simulink library "HDL_ieee_8021513"  (R2024a)
settings: Solver=FixedStepDiscrete  StartTime=0.0  StopTime=10.0  RelTol=1e-3
undefined symbols (not defined in the file or in its folder): Add, axiWidth, channelCyclicPrefixLen, channelDataCarriers, channelEstReference, channelLUT, channelOFDMSamples, channelScramblerInit, decimatorDelay, decimatorFilter, fPHY, frequencyOffsetTimeWindow, fs, headerBitsPerFec, headerBitsPerOFDMSymbol, headerBitsPerSubcarrier, headerCyclicPrefixLen, headerDataCarriers, headerOFDMSamples, headerScramblerInit, interpolatorDelay, interpolatorFilter, leftGuard, N, ncoCarrierFrequency, ncoWordLength, numDataCarriers, oversamplingFactor, payloadBitsPerFec, payloadScramblerInit, payloadWordsPerBlock0, peakDetectorThreshold, peakDetectorWindow, preambleCyclicPrefixLen, preambleDataCarriers, preambleLUT, preambleOFDMSamples, preambleScramblerInit, QAM, rightGuard, Shift
libraries: hdlsllib x198, $bdroot x80, whdlutilities x28, whdledac x10, whdlmod x7, simulink x4, dsphdlfiltering2 x2, dsphdlsigops2 x2, commhdlcrc x2, dspsigops x2, dspstat3 x2, commdigbbndam3 x2
(part 1 of 5)
settings Model: Creator=cotti  LastModifiedBy=cotti
settings OptimizationCC: BlockReduction=off  ConditionallyExecuteInputs=off  DefaultParameterBehavior=Inlined  InheritOutputTypeSmallerThanSingle=on  ReuseModelBlockBuffer=off
settings DebuggingCC: AlgebraicLoopMsg=error  SingleTaskRateTransMsg=error
settings HardwareCC: ProdBitPerPointer=32  ProdBitPerSizeT=32  ProdBitPerPtrDiffT=32  ProdLargestAtomicFloat=None  ProdIntDivRoundTo=Undefined  ProdEndianess=Unspecified  ProdWordSize=32  ProdHWDeviceType=ASIC/FPGA->ASIC/FPGA  TargetBitPerLong=64  TargetBitPerPointer=64  TargetBitPerSizeT=64  TargetBitPerPtrDiffT=64  TargetLongLongMode=on  TargetIntDivRoundTo=Zero  TargetEndianess=LittleEndian  TargetWordSize=64  TargetHWDeviceType=Custom Processor->MATLAB Host Computer  ProdEqTarget=off
settings RTWCC: GPUComputeCapability=3.5

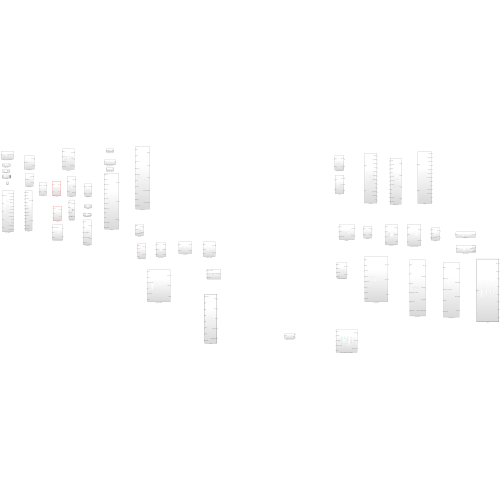
[thumbnail: Simulink's stored preview of the top-level diagram]
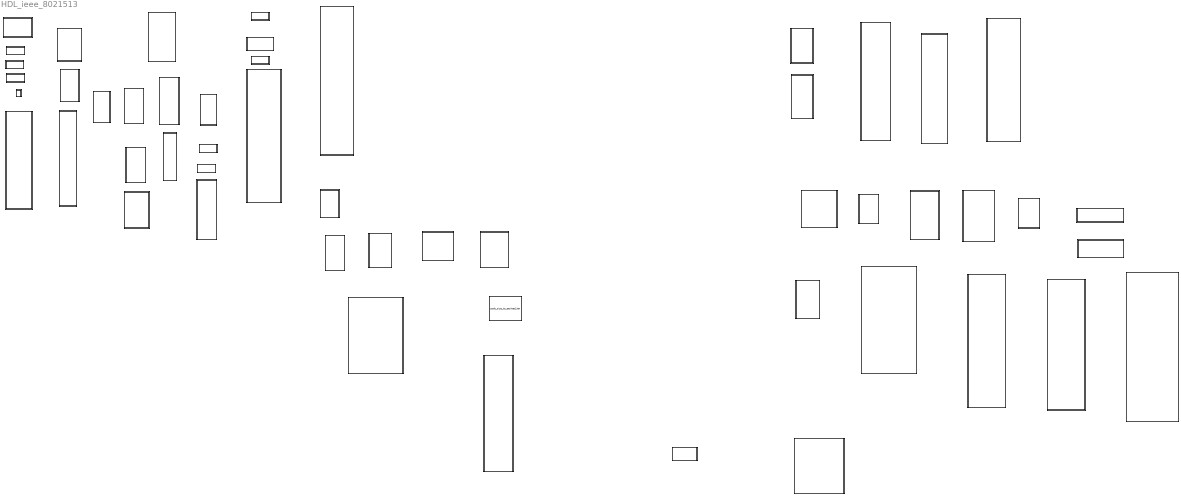
== system HDL_ieee_8021513 ==
  Buffer : Subsystem
  Deco_3a8 : Subsystem
  batid_to_bits_per_subcarrier : Subsystem
  calculate_mean_and_std : Subsystem
  channel_estimation_and_equalization : Subsystem
  channel_gen : Subsystem
  constellation_descrambler : Subsystem
  constellation_scrambler : Subsystem
  decimator : Subsystem
  downshifter : Subsystem
  falling_edge_detector : Subsystem
  frequency_upshift : Subsystem
  full_ofdm_modulator : Subsystem
  full_rx : Subsystem  TreatAsAtomicUnit=on
  full_tx : Subsystem  TreatAsAtomicUnit=on
  gnd_ctrl : Subsystem
  h_crc : Subsystem
  h_crc_rx : Subsystem
  h_gen : Subsystem
  h_remove_repetition : Subsystem
  h_repetition : Subsystem
  h_rx_full : Subsystem
  h_scrambler : Subsystem
      settings: LibrarySourceBlock=|
      | hdlsllib/Ports &
      | Subsystems/Subsystem
  h_separate : Subsystem
  header_fec : Subsystem
  header_full : Subsystem
      settings: LibrarySourceBlock=|
      | hdlsllib/Ports &
      | Subsystems/Subsystem
  interpolator : Subsystem
  ldpc_encoder : Subsystem
  next_frame_to_ready : Subsystem
  ofdm_demod : Subsystem
  ofdm_modulator : Subsystem
  ofdm_separator : Subsystem
  ofdm_symbol_sync : Subsystem
  p_scrambler : Subsystem
      settings: LibrarySourceBlock=|
      | hdlsllib/Ports &
      | Subsystems/Subsystem
  payload_full : Subsystem
  payload_rep : Subsystem
  peak_detector : Subsystem
  preamble_gen : Subsystem
  psdu_size_to_payload_len : $bdroot/payload_full/psdu_size_to_payload_len  SystemSampleTime=-1  VariantActivationTime=update diagram  AllowFlexibleInterface=on  Latency=0  AutoFrameSizeCalculation=off
  puncturer : Subsystem
  qam_demod : Subsystem
  qam_mod : Subsystem
  reduced_ldpc : Subsystem
  reg_to_variable : Subsystem
  remove_tone_mapping : Subsystem
  rising_edge_detector : Subsystem
  rx_demodulator_full : Subsystem
  rx_payload_full : Subsystem
  sync_constellation_scrambler : Subsystem
  tone_mapping : Subsystem
  valid_to_ctrl : Subsystem
  variable_to_reg : Subsystem

== system HDL_ieee_8021513/Buffer ==
  I : Inport
  O : Outport
  wires:
  I/1 -> O/1

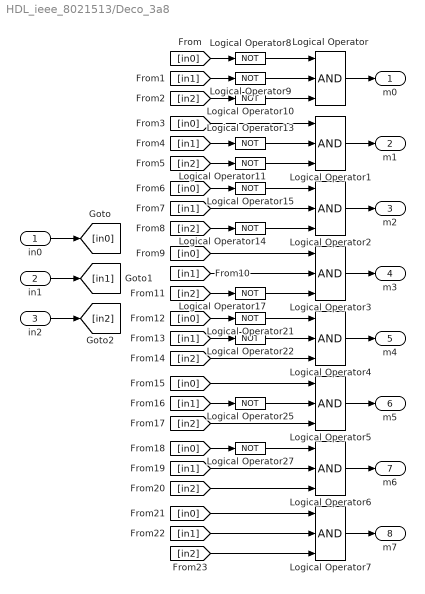
== system HDL_ieee_8021513/Deco_3a8 ==
  in0 : Inport
  in1 : Inport  Port=2
  in2 : Inport  Port=3
  Logical Operator{,1..7} (8 alike) : Logic  Inputs=3  IconShape=distinctive  AllPortsSameDT=off  OutDataTypeStr=boolean
  Logical Operator{8..11,13..15,17,21..22,25,27} (12 alike) : Logic  Operator=NOT  IconShape=distinctive  AllPortsSameDT=off  OutDataTypeStr=boolean
  m0 : Outport
  m1 : Outport  Port=2
  m2 : Outport  Port=3
  m3 : Outport  Port=4
  m4 : Outport  Port=5
  m5 : Outport  Port=6
  m6 : Outport  Port=7
  m7 : Outport  Port=8
  wires:
  Logical Operator/1 -> m0/1
  Logical Operator1/1 -> m1/1
  Logical Operator2/1 -> m2/1
  Logical Operator3/1 -> m3/1
  Logical Operator4/1 -> m4/1
  Logical Operator5/1 -> m5/1
  Logical Operator6/1 -> m6/1
  Logical Operator7/1 -> m7/1
  in0/1 -> [in0]
  in1/1 -> [in1]
  in2/1 -> [in2]
  [in0] -> Logical Operator8/1
  [in1] -> Logical Operator9/1
  [in2] -> Logical Operator10/1
  Logical Operator8/1 -> Logical Operator/1
  Logical Operator9/1 -> Logical Operator/2
  Logical Operator10/1 -> Logical Operator/3
  [in1] -> Logical Operator13/1
  [in2] -> Logical Operator11/1
  [in2] -> Logical Operator14/1
  [in0] -> Logical Operator15/1
  [in1] -> Logical Operator2/2
  [in2] -> Logical Operator17/1
  [in0] -> Logical Operator3/1
  [in1] -> Logical Operator3/2
  [in2] -> Logical Operator4/3
  [in0] -> Logical Operator21/1
  [in1] -> Logical Operator22/1
  [in2] -> Logical Operator5/3
  [in0] -> Logical Operator5/1
  [in1] -> Logical Operator25/1
  [in2] -> Logical Operator6/3
  [in0] -> Logical Operator27/1
  [in1] -> Logical Operator6/2
  [in2] -> Logical Operator7/3
  [in0] -> Logical Operator7/1
  [in1] -> Logical Operator7/2
  [in0] -> Logical Operator1/1
  Logical Operator13/1 -> Logical Operator1/2
  Logical Operator11/1 -> Logical Operator1/3
  Logical Operator15/1 -> Logical Operator2/1
  Logical Operator14/1 -> Logical Operator2/3
  Logical Operator22/1 -> Logical Operator4/2
  Logical Operator21/1 -> Logical Operator4/1
  Logical Operator17/1 -> Logical Operator3/3
  Logical Operator27/1 -> Logical Operator6/1
  Logical Operator25/1 -> Logical Operator5/2

== system HDL_ieee_8021513/batid_to_bits_per_subcarrier ==
  note: De momento, el valor de BATID va a coincidir con el valor de la cantidad de bits por subcarrier.
  note: Remember that "bat_id" is LSB first.
  bat_id : Inport
  Bit Concat : hdlsllib/Logic and Bit Operations/Bit Concat  numInputs=4
  Demux : Demux  Outputs=5
  Terminator : Terminator
  bits_per_subcarrier : Outport
  wires:
  bat_id/1 -> Demux/1
  Demux/3 -> [bat2]
  Demux/2 -> [bat1]
  Demux/4 -> [bat3]
  Demux/5 -> Terminator/1
  Demux/1 -> [bat0]
  Bit Concat/1 -> bits_per_subcarrier/1
  [bat3] -> Bit Concat/1
  [bat2] -> Bit Concat/2
  [bat1] -> Bit Concat/3
  [bat0] -> Bit Concat/4

== system HDL_ieee_8021513/calculate_mean_and_std ==
  data_in : Inport
  Delay{6..8,10..11} (5 alike) : Delay  DelayLength=1  InitialCondition=0  UseCircularBuffer=on
  Square : Math  Operator=square  SignedPower=on  RndMeth=Zero
  Subtract : Sum  Inputs=+-  OutDataTypeStr=Inherit: Same as first input
  calculate_mean_x : Subsystem
  calculate_mean_x_squared : Subsystem
  multiply by 2 : hdlsllib/Logic and Bit Operations/Bit Shift  mode=Shift Left Logical  N=1
  std : Outport
  mean : Outport  Port=2
  wires:
  Delay11/1 -> mean/1
  Subtract/1 -> Delay8/1
  Delay10/1 -> Delay11/1
  Square/1 -> Delay7/1
  Delay8/1 -> multiply by 2/1
  Delay6/1 -> Subtract/1
  calculate_mean_x/1(mean) -> Delay10/1, Square/1
  Delay7/1 -> Subtract/2
  calculate_mean_x_squared/1(mean_x_squared) -> Delay6/1
  data_in/1 -> calculate_mean_x/1(data_in), calculate_mean_x_squared/1(data_in)
  multiply by 2/1 -> std/1

== system HDL_ieee_8021513/channel_estimation_and_equalization ==
  note: Stores the estimate from Channel Estimation subsystem for each frame and perform channel equalization.
  note: Estimates the channel frequency response for each frame.
  data_in : Inport
  valid_data : Inport  Port=2
  valid_channel : Inport  Port=3
  dont_use_equalizer : Inport  Port=4
  reset : Inport  Port=5
  Channel Equalization : Subsystem
  Channel Estimation : Subsystem
  Delay{1..6,10..11,13..14} (10 alike) : Delay  DelayLength=1  InitialCondition=0
  Delay21 : Delay  InitialCondition=0
  Delay22 : Delay  InitialCondition=0
  data_out : Outport
  valid_out : Outport  Port=2
  channel_est_out : Outport  Port=3
  wires:
  reset/1 -> Channel Estimation/3(reset), Channel Equalization/6(reset)
  Delay4/1 -> channel_est_out/1
  Channel Equalization/3(channel_est_out) -> Delay4/1
  Channel Estimation/1(channel_estimate) -> Delay13/1  "channelEstimates"
  Delay22/1 -> Delay11/1
  Delay21/1 -> Delay10/1
  valid_channel/1 -> Delay2/1
  data_in/1 -> Delay1/1
  valid_data/1 -> Delay3/1
  Delay2/1 -> Channel Estimation/2(valid_in)
  Channel Estimation/2(valid_estimate) -> Delay14/1  "channelEstimatesValid"
  Delay3/1 -> Delay22/1
  Delay1/1 -> Channel Estimation/1(data_in), Delay21/1
  Channel Equalization/2(valid_out) -> Delay6/1
  Channel Equalization/1(data_out) -> Delay5/1
  Delay10/1 -> Channel Equalization/1(data_in)
  Delay11/1 -> Channel Equalization/2(valid_data)
  Delay13/1 -> Channel Equalization/3(channel_estimate_in)
  Delay14/1 -> Channel Equalization/4(valid_channel_estimate)
  Delay6/1 -> valid_out/1
  dont_use_equalizer/1 -> Channel Equalization/5(dont_use_equalizer)
  Delay5/1 -> data_out/1

== system HDL_ieee_8021513/channel_gen ==
  new_frame : Inport
  Delay : Delay  DelayLength=1  InitialCondition=0  UseCircularBuffer=on
  Direct Lookup Table (n-D) : LookupNDDirect  NumberOfTableDimensions=1  Table=channelLUT  DiagnosticForOutOfRangeInput=Error  RemoveProtectionInput=on  TableDataTypeStr=boolean
  HDL Counter : hdlsllib/Sources/HDL Counter  CountType=Count limited  CountInit=0  CountStep=1  CountMax=length(channelLUT)-1  CountFromType=Initial value  CountFrom=0  CountResetPort=off  CountLoadPort=off  CountEnbPort=on  CountDirPort=off  CountHitOutputPort=on  CountDataType=Unsigned  CountWordLen=9  CountFracLen=0  CountSampTime=1
  Logical Operator : Logic  Operator=NOT  IconShape=distinctive  AllPortsSameDT=off  OutDataTypeStr=boolean
  Logical Operator1 : Logic  Operator=OR  IconShape=distinctive  AllPortsSameDT=off  OutDataTypeStr=boolean
  Unit Delay Enabled Synchronous : hdlsllib/Discrete/Unit Delay Enabled Synchronous  InitialCondition=0.0  SampleTime=-1
  valid_to_ctrl : $bdroot/valid_to_ctrl  SystemSampleTime=-1  VariantActivationTime=update diagram  AllowFlexibleInterface=on  Latency=0  AutoFrameSizeCalculation=off
  data_out : Outport
  ctrl_out : Outport  Port=2
  wires:
  Unit Delay Enabled Synchronous/1 -> HDL Counter/1, valid_to_ctrl/1
  HDL Counter/1 -> Direct Lookup Table (n-D)/1
  Logical Operator/1 -> Unit Delay Enabled Synchronous/1
  Direct Lookup Table (n-D)/1 -> Delay/1
  valid_to_ctrl/1 -> ctrl_out/1
  Delay/1 -> data_out/1
  new_frame/1 -> Logical Operator1/1
  HDL Counter/2 -> Logical Operator1/2, Logical Operator/1
  Logical Operator1/1 -> Unit Delay Enabled Synchronous/2

== system HDL_ieee_8021513/constellation_descrambler ==
  data_in : Inport
  valid_in : Inport  Port=2
  init : Inport  Port=3
  rising_edge_detector : $bdroot/rising_edge_detector  SystemSampleTime=-1  VariantActivationTime=update diagram  AllowFlexibleInterface=on  Latency=0  AutoFrameSizeCalculation=off
  rotate_-90 : Subsystem
  sync_constellation_scrambler : $bdroot/sync_constellation_scrambler  SystemSampleTime=-1  VariantActivationTime=update diagram  AllowFlexibleInterface=on  Latency=0  AutoFrameSizeCalculation=off
  data_out : Outport
  valid_out : Outport  Port=2
  wires:
  rotate_-90/1(data_out) -> data_out/1
  rotate_-90/2(valid_out) -> valid_out/1
  sync_constellation_scrambler/2 -> rotate_-90/4(s2_in)  "s2"
  sync_constellation_scrambler/1 -> rotate_-90/3(s1_in)  "s1"
  valid_in/1 -> sync_constellation_scrambler/3, rotate_-90/2(valid_in), rising_edge_detector/1  "valid"
  init/1 -> sync_constellation_scrambler/2
  data_in/1 -> rotate_-90/1(data_in)
  rising_edge_detector/1 -> sync_constellation_scrambler/1  "start"

== system HDL_ieee_8021513/constellation_scrambler ==
  data_in : Inport
  valid_in : Inport  Port=2
  s1_in : Inport  Port=3
  s2_in : Inport  Port=4
  Delay : Delay  InitialCondition=0  UseCircularBuffer=on
  Delay1 : Delay  InitialCondition=0  UseCircularBuffer=on
  Delay2 : Delay  DelayLength=1  InitialCondition=0  UseCircularBuffer=on
  Delay3 : Delay  DelayLength=1  InitialCondition=0  UseCircularBuffer=on
  rotate : Subsystem
  data_out : Outport  VectorParamsAs1DForOutWhenUnconnected=off
  valid_out : Outport  Port=2  VectorParamsAs1DForOutWhenUnconnected=off
  wires:
  valid_in/1 -> Delay1/1  "en"
  data_in/1 -> Delay/1
  Delay/1 -> rotate/3(data_in)  "data_in"
  rotate/1(data_out) -> Delay2/1  "data_out"
  Delay1/1 -> Delay3/1
  Delay2/1 -> data_out/1  "data_out"
  Delay3/1 -> valid_out/1
  s1_in/1 -> rotate/2(s1)  "s1"
  s2_in/1 -> rotate/1(s2)  "s2"

== system HDL_ieee_8021513/decimator ==
  note: The data out from this blocks is "valid" one sample, and invalid the next.
      | This blocks makes sure that the data is valid both cycles.
      | What happens is that the ZOH might sample the signal when is valid or invalid.
  data_in : Inport
  valid_in : Inport  Port=2
  Delay{,4..7} (5 alike) : Delay  DelayLength=1  InitialCondition=0  UseCircularBuffer=on
  Delay1 : Delay  DelayLength=decimatorDelay/2  InitialCondition=0  UseCircularBuffer=on
  Delay3 : Delay  DelayLength=(decimatorDelay)*3 + 6  InitialCondition=0  UseCircularBuffer=on
  FIR Decimator : dsphdlfiltering2/FIR Decimator  Numerator=decimatorFilter.Numerator  FilterStructure=Direct form systolic  DecimationFactor=oversamplingFactor  NumCycles=1  SimulateUsing=Code generation  roundingMode=Floor  overflowMode=off  CoefficientsDataTypeStr=fixdt(1,16)  OutputDataTypeStr=fixdt(1,16,12)  ResetInputPort=off  HDLGlobalReset=off
  Logical Operator : Logic  Operator=OR  IconShape=distinctive  AllPortsSameDT=off  OutDataTypeStr=boolean
  Logical Operator1 : Logic  IconShape=distinctive  AllPortsSameDT=off  OutDataTypeStr=boolean
  Logical Operator2 : Logic  IconShape=distinctive  AllPortsSameDT=off  OutDataTypeStr=boolean
  Logical Operator3 : Logic  Operator=NOT  IconShape=distinctive  AllPortsSameDT=off  OutDataTypeStr=boolean
  Rate Transition : RateTransition  OutPortSampleTimeOpt=Multiple of input port sample time  OutPortSampleTimeMultiple=oversamplingFactor
  Rate Transition1 : RateTransition  OutPortSampleTimeOpt=Multiple of input port sample time  OutPortSampleTimeMultiple=oversamplingFactor
  Switch : Switch  Criteria=u2 ~= 0  SaturateOnIntegerOverflow=off  InputSameDT=off
  Switch1 : Switch  Criteria=u2 ~= 0  SaturateOnIntegerOverflow=off  InputSameDT=off
  falling_edge_detector : $bdroot/falling_edge_detector  SystemSampleTime=-1  VariantActivationTime=update diagram  AllowFlexibleInterface=on  Latency=0  AutoFrameSizeCalculation=off
  data_out : Outport
  valid_out : Outport  Port=2
  wires:
  Delay5/1 -> FIR Decimator/1
  Rate Transition/1 -> Delay1/1, Logical Operator1/1
  Delay4/1 -> data_out/1
  falling_edge_detector/1 -> Logical Operator3/1
  Logical Operator2/1 -> valid_out/1
  Logical Operator1/1 -> falling_edge_detector/1, Delay/1
  Logical Operator3/1 -> Logical Operator2/2
  Delay/1 -> Logical Operator2/1
  Delay7/1 -> Switch1/3
  Delay6/1 -> Switch/3
  FIR Decimator/2 -> Switch1/2, Switch1/1, Switch/2, Delay7/1  "valid_out"
  Switch1/1 -> Rate Transition/1
  FIR Decimator/1 -> Delay6/1, Switch/1  "data_out"
  Switch/1 -> Rate Transition1/1
  data_in/1 -> Delay5/1  "data_in"
  Logical Operator/1 -> FIR Decimator/2
  Delay3/1 -> Logical Operator/2
  Delay1/1 -> Logical Operator1/2
  Rate Transition1/1 -> Delay4/1
  valid_in/1 -> Delay3/1, Logical Operator/1

== system HDL_ieee_8021513/downshifter ==
  data_in : Inport
  valid_in : Inport  Port=2
  frequency_offset : Inport  Port=3
  Add : Sum  OutDataTypeStr=Inherit: Same as first input
  Constant : Constant  Value=ncoCarrierFrequency  OutDataTypeStr=int32  SampleTime=1/fs
  Delay : Delay  DelayLength=6  InitialCondition=0  UseCircularBuffer=on
  Delay1 : Delay  DelayLength=4  InitialCondition=0  UseCircularBuffer=on
  Delay{2..3,5..8} (6 alike) : Delay  DelayLength=1  InitialCondition=0  UseCircularBuffer=on
  Gain : Gain  Gain=fi(2^ncoWordLength/fs, 0, 32, 32)  ParamDataTypeStr=fixdt(0,32,32)  OutDataTypeStr=uint32  RndMeth=Round
  NCO : dsphdlsigops2/NCO  PhaseIncrementSource=Input port  PhaseIncrement=ncoPhaseIncrement  PhaseOffsetSource=Property  PhaseOffset=0  DitherSource=None  NumDitherBits=1  SamplesPerFrame=1  LUTCompress=off  ResetAction=on  Waveform=Complex exponential  PhasePort=off  SimulateUsing=Code generation  AccumulatorWL=ncoWordLength  PhaseQuantization=on  NumQuantizerAccumulatorBits=ncoQuantization  OutputDataType=Binary point scaling  OutputWL=16  OutputFL=12
  digital_carrier_receiver : Subsystem
  rising_edge_detector : $bdroot/rising_edge_detector  SystemSampleTime=-1  VariantActivationTime=update diagram  AllowFlexibleInterface=on  Latency=0  AutoFrameSizeCalculation=off
  data_out : Outport  VectorParamsAs1DForOutWhenUnconnected=off
  valid_out : Outport  Port=2  VectorParamsAs1DForOutWhenUnconnected=off
  wires:
  valid_in/1 -> Delay7/1
  Delay1/1 -> valid_out/1
  NCO/2 -> Delay1/1
  Delay3/1 -> Delay/1
  digital_carrier_receiver/1(data_out) -> data_out/1
  NCO/1 -> digital_carrier_receiver/2(ncoIn)
  Delay/1 -> digital_carrier_receiver/1(dataIn)
  data_in/1 -> Delay8/1
  Delay2/1 -> NCO/3  "valid"
  rising_edge_detector/1 -> NCO/2
  Constant/1 -> Add/1
  Add/1 -> Delay6/1
  Delay5/1 -> NCO/1  "inc"
  Delay6/1 -> Gain/1
  Gain/1 -> Delay5/1
  Delay7/1 -> rising_edge_detector/1, Delay2/1
  Delay8/1 -> Delay3/1
  frequency_offset/1 -> Add/2

== system HDL_ieee_8021513/falling_edge_detector ==
  in : Inport
  Delay : Delay  DelayLength=1  InitialCondition=0  UseCircularBuffer=on
  Logical Operator : Logic  IconShape=distinctive  AllPortsSameDT=off  OutDataTypeStr=boolean
  Logical Operator1 : Logic  Operator=NOT  IconShape=distinctive  AllPortsSameDT=off  OutDataTypeStr=boolean
  out : Outport  VectorParamsAs1DForOutWhenUnconnected=off
  wires:
  in/1 -> Logical Operator1/1, Delay/1
  Delay/1 -> Logical Operator/2
  Logical Operator/1 -> out/1
  Logical Operator1/1 -> Logical Operator/1

== system HDL_ieee_8021513/frequency_upshift ==
  data_in : Inport
  valid_in : Inport  Port=2
  reset : Inport  Port=3
  Delay : Delay  DelayLength=6  InitialCondition=0  UseCircularBuffer=on
  Delay1 : Delay  DelayLength=4  InitialCondition=0  UseCircularBuffer=on
  Delay2 : Delay  DelayLength=1  InitialCondition=0  UseCircularBuffer=on
  Delay3 : Delay  DelayLength=1  InitialCondition=0  UseCircularBuffer=on
  Mixer : Subsystem
  NCO : dsphdlsigops2/NCO  PhaseIncrementSource=Property  PhaseIncrement=ncoUpshifterPhaseIncrement  PhaseOffsetSource=Property  PhaseOffset=0  DitherSource=None  NumDitherBits=1  SamplesPerFrame=1  LUTCompress=off  ResetAction=on  Waveform=Complex exponential  PhasePort=off  SimulateUsing=Code generation  AccumulatorWL=ncoUpshifterWordLength  PhaseQuantization=off  NumQuantizerAccumulatorBits=6  OutputDataType=Binary point scaling  OutputWL=16  OutputFL=14
  data_out : Outport  VectorParamsAs1DForOutWhenUnconnected=off
  valid_out : Outport  Port=2  VectorParamsAs1DForOutWhenUnconnected=off
  wires:
  Delay2/1 -> NCO/2
  reset/1 -> NCO/1
  Delay3/1 -> Delay/1
  data_in/1 -> Delay3/1
  valid_in/1 -> Delay2/1
  NCO/1 -> Mixer/2(ncoIn)
  Mixer/1(mixedOut) -> data_out/1
  Delay/1 -> Mixer/1(dataIn)
  NCO/2 -> Delay1/1
  Delay1/1 -> valid_out/1

== system HDL_ieee_8021513/full_ofdm_modulator ==
  data_in : Inport
  valid_in : Inport  Port=2
  bits_per_subcarrier : Inport  Port=3
  init : Inport  Port=4
  new_ofdm_sym : Inport  Port=5
  cp_len : Inport  Port=6
  Delay1 : Delay  DelayLength=1  InitialCondition=0  UseCircularBuffer=on
  Logical Operator : Logic  IconShape=distinctive  AllPortsSameDT=off  OutDataTypeStr=boolean
  Logical Operator3 : Logic  IconShape=distinctive  AllPortsSameDT=off  OutDataTypeStr=boolean
  enabled_qam_and_scrambler : Subsystem  TreatAsAtomicUnit=on
  frequency_upshift : $bdroot/frequency_upshift  SystemSampleTime=-1  VariantActivationTime=update diagram  AllowFlexibleInterface=on  Latency=0  AutoFrameSizeCalculation=off
  interpolator : $bdroot/interpolator  SystemSampleTime=-1  VariantActivationTime=update diagram  AllowFlexibleInterface=on  Latency=0  AutoFrameSizeCalculation=off
  ofdm_modulator : $bdroot/ofdm_modulator  SystemSampleTime=-1  VariantActivationTime=update diagram  AllowFlexibleInterface=on  Latency=0  AutoFrameSizeCalculation=off
  rising_edge_detector : $bdroot/rising_edge_detector  SystemSampleTime=-1  VariantActivationTime=update diagram  AllowFlexibleInterface=on  Latency=0  AutoFrameSizeCalculation=off
  sync_constellation_scrambler : $bdroot/sync_constellation_scrambler  SystemSampleTime=-1  VariantActivationTime=update diagram  AllowFlexibleInterface=on  Latency=0  AutoFrameSizeCalculation=off
  data_out : Outport  VectorParamsAs1DForOutWhenUnconnected=off
  valid_out : Outport  Port=2  VectorParamsAs1DForOutWhenUnconnected=off
  ready : Outport  Port=3  VectorParamsAs1DForOutWhenUnconnected=off
  wires:
  enabled_qam_and_scrambler/4(valid_scrambler) -> Logical Operator/1
  enabled_qam_and_scrambler/6(new_out) -> sync_constellation_scrambler/1
  enabled_qam_and_scrambler/5(init_out) -> sync_constellation_scrambler/2
  enabled_qam_and_scrambler/3(cp_len_out) -> ofdm_modulator/3
  sync_constellation_scrambler/2 -> enabled_qam_and_scrambler/7(s2_in)
  sync_constellation_scrambler/1 -> enabled_qam_and_scrambler/8(s1_in)
  Logical Operator/1 -> sync_constellation_scrambler/3
  Logical Operator3/1 -> ofdm_modulator/2  "valid_new"
  enabled_qam_and_scrambler/1(data_out) -> ofdm_modulator/1  "out_new"
  Delay1/1 -> enabled_qam_and_scrambler/Enable, ready/1, Logical Operator3/1  "ready_out"
  data_in/1 -> enabled_qam_and_scrambler/1(data_in)
  init/1 -> enabled_qam_and_scrambler/4(init)
  enabled_qam_and_scrambler/2(valid_out) -> Logical Operator3/2
  ofdm_modulator/3 -> Delay1/1, Logical Operator/2
  ofdm_modulator/2 -> interpolator/2
  frequency_upshift/1 -> data_out/1
  frequency_upshift/2 -> valid_out/1
  new_ofdm_sym/1 -> enabled_qam_and_scrambler/5(new)
  bits_per_subcarrier/1 -> enabled_qam_and_scrambler/3(bits_per_subcarrier)
  interpolator/2 -> rising_edge_detector/1, frequency_upshift/2
  valid_in/1 -> enabled_qam_and_scrambler/2(valid_in)
  ofdm_modulator/1 -> interpolator/1
  interpolator/1 -> frequency_upshift/1
  rising_edge_detector/1 -> frequency_upshift/3
  cp_len/1 -> enabled_qam_and_scrambler/6(cp_len)

== system HDL_ieee_8021513/full_rx ==
  data_in : Inport
  Data Type Conversion : DataTypeConversion  OutDataTypeStr=fixdt(1,16,12)  SaturateOnIntegerOverflow=off  RndMeth=Floor
  Rate Transition{,1..2,9} (4 alike) : RateTransition  OutPortSampleTime=1/fPHY
  Rate Transition{5..8} (4 alike) : RateTransition  OutPortSampleTime=1/(4*fPHY)
  Terminator1 : Terminator
  batid_to_bits_per_subcarrier : $bdroot/batid_to_bits_per_subcarrier  SystemSampleTime=-1  VariantActivationTime=update diagram  AllowFlexibleInterface=on  Latency=0  AutoFrameSizeCalculation=off
  cpid_to_cplen : Subsystem
  h_rx_full : $bdroot/h_rx_full  SystemSampleTime=-1  VariantActivationTime=update diagram  AllowFlexibleInterface=on  Latency=0  AutoFrameSizeCalculation=off
  header_clock_x2 : Subsystem
  prepare_payload_data : Subsystem
  rx_demodulator_full : $bdroot/rx_demodulator_full  SystemSampleTime=-1  VariantActivationTime=update diagram  AllowFlexibleInterface=on  Latency=0  AutoFrameSizeCalculation=off
  rx_payload_full : $bdroot/rx_payload_full  SystemSampleTime=-1  VariantActivationTime=update diagram  AllowFlexibleInterface=on  Latency=0  AutoFrameSizeCalculation=off
  variable_to_reg : $bdroot/variable_to_reg  SystemSampleTime=-1  VariantActivationTime=update diagram  AllowFlexibleInterface=on  Latency=0  AutoFrameSizeCalculation=off
  data_out : Outport
  valid_out : Outport  Port=2
  reg0 : Outport  Port=3
  reg1 : Outport  Port=4
  reg2 : Outport  Port=5
  reg3 : Outport  Port=6
  end : Outport  Port=7
  err : Outport  Port=8
  wires:
  rx_demodulator_full/3 -> prepare_payload_data/2(valid_payload)  "valid_payload"
  rx_demodulator_full/2 -> header_clock_x2/2(valid_header)  "valid_header"
  Rate Transition9/1 -> rx_demodulator_full/5
  Rate Transition/1 -> rx_demodulator_full/4
  Rate Transition1/1 -> rx_demodulator_full/3
  Rate Transition2/1 -> rx_demodulator_full/2
  h_rx_full/6 -> variable_to_reg/6
  batid_to_bits_per_subcarrier/1 -> [payloadBitsPerSubcarrier]
  Rate Transition7/1 -> rx_payload_full/7
  variable_to_reg/1 -> reg0/1  "reg0"
  prepare_payload_data/3(last_frame) -> rx_payload_full/3
  header_clock_x2/2(start) -> h_rx_full/2
  rx_payload_full/3 -> [payloadReady]
  cpid_to_cplen/1(payload_cp_len) -> [payloadCpLen]
  h_rx_full/10 -> variable_to_reg/10
  Rate Transition5/1 -> rx_payload_full/5
  Rate Transition6/1 -> rx_payload_full/6
  h_rx_full/5 -> variable_to_reg/5
  data_in/1 -> rx_demodulator_full/1
  h_rx_full/4 -> variable_to_reg/4, Rate Transition6/1
  rx_demodulator_full/1 -> Data Type Conversion/1
  prepare_payload_data/1(dataOut) -> rx_payload_full/1
  h_rx_full/3 -> variable_to_reg/3, Rate Transition7/1
  Data Type Conversion/1 -> header_clock_x2/1(data_in), prepare_payload_data/1(data_in)
  Rate Transition8/1 -> rx_payload_full/8
  h_rx_full/11 -> variable_to_reg/11
  [payloadReady] -> prepare_payload_data/3(payload_ready)  "payload_ready"
  rx_payload_full/1 -> data_out/1
  h_rx_full/8 -> batid_to_bits_per_subcarrier/1, variable_to_reg/8
  rx_payload_full/2 -> valid_out/1
  h_rx_full/1 -> Rate Transition8/1, [psduSize], variable_to_reg/1
  h_rx_full/2 -> variable_to_reg/2
  h_rx_full/9 -> cpid_to_cplen/1(cp_id), variable_to_reg/9
  prepare_payload_data/2(valid_in) -> rx_payload_full/2  "valid_payload_to_ldpc"
  [psduSize] -> Rate Transition/1
  [payloadCpLen] -> Rate Transition2/1
  h_rx_full/13 -> err/1
  prepare_payload_data/4(new_frame) -> rx_payload_full/4
  h_rx_full/7 -> variable_to_reg/7, Rate Transition5/1
  [payloadBitsPerSubcarrier] -> Rate Transition1/1
  header_clock_x2/1(data_out) -> h_rx_full/1
  variable_to_reg/4 -> reg3/1  "reg3"
  variable_to_reg/2 -> reg1/1  "reg1"
  variable_to_reg/3 -> reg2/1  "reg2"
  h_rx_full/12 -> end/1, [header_end]  "header_ready"
  [header_end] -> Rate Transition9/1
  rx_demodulator_full/4 -> Terminator1/1  "last_frame"

== system HDL_ieee_8021513/full_tx ==
  new_frame_in : Inport
  reg0 : Inport  Port=2
  reg1 : Inport  Port=3
  reg2 : Inport  Port=4
  reg3 : Inport  Port=5
  data_in : Inport  Port=6
  valid_in : Inport  Port=7
  last_frame : Inport  Port=8
  Delay1 : Delay  DelayLength=1  InitialCondition=0  UseCircularBuffer=on
  FIFO : Subsystem  Commented=on
  Rate Transition : RateTransition  OutPortSampleTime=1/fPHY
  Sample Control Bus Selector : whdlutilities/Sample Control Bus Selector  OutputSignals=start,end,valid
  Terminator : Terminator
  Terminator1 : Terminator
  Terminator2 : Terminator
  channel_gen : $bdroot/channel_gen  SystemSampleTime=-1  VariantActivationTime=update diagram  AllowFlexibleInterface=on  Latency=0  AutoFrameSizeCalculation=off
  clock_crossing : Subsystem
  full_ofdm_modulator : $bdroot/full_ofdm_modulator  SystemSampleTime=-1  VariantActivationTime=update diagram  AllowFlexibleInterface=on  Latency=0  AutoFrameSizeCalculation=off
  header_full : $bdroot/header_full  SystemSampleTime=-1  VariantActivationTime=update diagram  AllowFlexibleInterface=on  Latency=0  AutoFrameSizeCalculation=off
      settings: LibrarySourceBlock=|
      | hdlsllib/Ports &
      | Subsystems/Subsystem
  new_frame_rate_conversion : Subsystem
  new_frame_rate_conversion1 : Subsystem
  payload_full : $bdroot/payload_full  SystemSampleTime=-1  VariantActivationTime=update diagram  AllowFlexibleInterface=on  Latency=0  AutoFrameSizeCalculation=off
  preamble_gen : $bdroot/preamble_gen  SystemSampleTime=-1  VariantActivationTime=update diagram  AllowFlexibleInterface=on  Latency=0  AutoFrameSizeCalculation=off
  reg_to_variable : $bdroot/reg_to_variable  SystemSampleTime=-1  VariantActivationTime=update diagram  AllowFlexibleInterface=on  Latency=0  AutoFrameSizeCalculation=off
  store_frame_in_ram : Subsystem
  data_out : Outport
  valid_out : Outport  Port=2
  ready : Outport  Port=3
  debug_payload : Outport  Port=4  VectorParamsAs1DForOutWhenUnconnected=off
  debug_payload_ctrl : Outport  Port=5  VectorParamsAs1DForOutWhenUnconnected=off
  wires:
  full_ofdm_modulator/3 -> store_frame_in_ram/12(ready)  "ready"
  store_frame_in_ram/6(cp_len) -> full_ofdm_modulator/6
  store_frame_in_ram/5(new) -> full_ofdm_modulator/5
  store_frame_in_ram/4(init) -> full_ofdm_modulator/4
  store_frame_in_ram/3(bits_per_subcarrier_out) -> full_ofdm_modulator/3
  store_frame_in_ram/2(valid_out) -> full_ofdm_modulator/2
  store_frame_in_ram/1(data_out) -> full_ofdm_modulator/1
  clock_crossing/1(preamble_out) -> store_frame_in_ram/1(preamble)
  clock_crossing/2(preamble_valid) -> store_frame_in_ram/2(preamble_valid)
  clock_crossing/3(channel_out) -> store_frame_in_ram/3(channel)
  clock_crossing/4(channel_valid) -> store_frame_in_ram/4(channel_valid)
  clock_crossing/5(header_out) -> store_frame_in_ram/5(header)
  clock_crossing/6(header_valid) -> store_frame_in_ram/6(header_valid)
  clock_crossing/7(payload_out) -> store_frame_in_ram/7(payload)
  clock_crossing/8(payload_valid_out) -> store_frame_in_ram/8(payload_valid)
  clock_crossing/9(payload_len_out) -> store_frame_in_ram/9(payload_len)
  clock_crossing/10(bits_per_subcarrier_out) -> store_frame_in_ram/10(bits_per_subcarrier)
  clock_crossing/11(cp_len_out) -> store_frame_in_ram/11(cp_len_in)
  Sample Control Bus Selector/2 -> channel_gen/1
  Sample Control Bus Selector/3 -> Terminator/1
  payload_full/1 -> debug_payload/1, clock_crossing/7(payload_in)
  reg_to_variable/3 -> header_full/3
  channel_gen/2 -> new_frame_rate_conversion/1(ctrl_in), clock_crossing/4(channel_ctrl)
  payload_full/5 -> clock_crossing/11(bits_per_subcarrier_in)
  reg_to_variable/9 -> payload_full/8, header_full/9
  reg_to_variable/11 -> header_full/11
  header_full/2 -> new_frame_rate_conversion1/1(ctrl_in), clock_crossing/6(header_ctrl_in)
  Rate Transition/1 -> preamble_gen/1
  header_full/1 -> clock_crossing/5(header_in)
  reg_to_variable/8 -> payload_full/5, header_full/8
  header_full/3 -> Terminator2/1
  reg_to_variable/10 -> clock_crossing/9(cp_len_in), header_full/10
  reg_to_variable/6 -> payload_full/10, header_full/6
  valid_in/1 -> payload_full/2
  channel_gen/1 -> clock_crossing/3(channel)
  new_frame_in/1 -> reg_to_variable/1
  new_frame_rate_conversion/1(new_frame) -> header_full/1
  preamble_gen/1 -> clock_crossing/1(preamble_in)
  reg1/1 -> reg_to_variable/3
  full_ofdm_modulator/2 -> valid_out/1  "valid_out"
  reg3/1 -> reg_to_variable/5
  last_frame/1 -> Delay1/1
  preamble_gen/2 -> clock_crossing/2(preamble_ctrl_in), Sample Control Bus Selector/1
  reg_to_variable/12 -> header_full/12
  new_frame_rate_conversion1/1(new_frame) -> payload_full/4  "payload_new_frame_in"
  reg2/1 -> reg_to_variable/4
  reg_to_variable/2 -> payload_full/9, header_full/2
  reg_to_variable/5 -> payload_full/6, header_full/5
  payload_full/3 -> ready/1
  payload_full/4 -> clock_crossing/10(payload_len_in)
  reg_to_variable/1 -> Rate Transition/1
  reg_to_variable/7 -> header_full/7
  data_in/1 -> payload_full/1
  Sample Control Bus Selector/1 -> Terminator1/1
  full_ofdm_modulator/1 -> data_out/1
  reg0/1 -> reg_to_variable/2
  payload_full/2 -> clock_crossing/8(payload_ctrl_in), debug_payload_ctrl/1  "payload_ctrl_out"
  reg_to_variable/4 -> payload_full/7, header_full/4
  Delay1/1 -> payload_full/3

== system HDL_ieee_8021513/gnd_ctrl ==
  Ground : Ground
  Ground1 : Ground
  Ground2 : Ground
  Sample Control Bus Creator : whdlutilities/Sample Control Bus Creator
  gnd_ctrl : Outport
  wires:
  Ground/1 -> Sample Control Bus Creator/3
  Ground1/1 -> Sample Control Bus Creator/2
  Ground2/1 -> Sample Control Bus Creator/1
  Sample Control Bus Creator/1 -> gnd_ctrl/1

== system HDL_ieee_8021513/h_crc ==
  data_in : Inport
  ctrl_in : Inport  Port=2
  General CRC Generator HDL Optimized : commhdlcrc/General CRC Generator HDL Optimized  Polynomial=headerCRCPoly  InitialState=1  DirectMethod=on  ReflectInput=off  ReflectCRCChecksum=off  FinalXORValue=0  SimulateUsing=Code generation
  Sample Control Bus Creator : whdlutilities/Sample Control Bus Creator
  Sample Control Bus Selector : whdlutilities/Sample Control Bus Selector  OutputSignals=start,end,valid
  data_out : Outport
  ctrl_out : Outport  Port=2
  wires:
  Sample Control Bus Creator/1 -> ctrl_out/1
  General CRC Generator HDL Optimized/2 -> Sample Control Bus Creator/1
  General CRC Generator HDL Optimized/3 -> Sample Control Bus Creator/2
  General CRC Generator HDL Optimized/4 -> Sample Control Bus Creator/3
  General CRC Generator HDL Optimized/1 -> data_out/1
  data_in/1 -> General CRC Generator HDL Optimized/1
  ctrl_in/1 -> Sample Control Bus Selector/1
  Sample Control Bus Selector/1 -> General CRC Generator HDL Optimized/2
  Sample Control Bus Selector/2 -> General CRC Generator HDL Optimized/3
  Sample Control Bus Selector/3 -> General CRC Generator HDL Optimized/4

== system HDL_ieee_8021513/h_crc_rx ==
  data_in : Inport
  ctrl_in : Inport  Port=2
  General CRC Syndrome Detector HDL Optimized : commhdlcrc/General CRC Syndrome Detector HDL Optimized  Polynomial=headerCRCPoly  InitialState=1  DirectMethod=on  ReflectInput=off  ReflectCRCChecksum=off  FinalXORValue=0  SimulateUsing=Code generation
  Sample Control Bus Creator : whdlutilities/Sample Control Bus Creator
  Sample Control Bus Selector : whdlutilities/Sample Control Bus Selector  OutputSignals=start,end,valid
  Switch : Switch  Criteria=u2 ~= 0  SaturateOnIntegerOverflow=off  InputSameDT=off
  Unit Delay : UnitDelay  SampleTime=-1  HasFrameUpgradeWarning=on
  data_out : Outport
  ctrl_out : Outport  Port=2  VectorParamsAs1DForOutWhenUnconnected=off
  err : Outport  Port=3  VectorParamsAs1DForOutWhenUnconnected=off
  wires:
  ctrl_in/1 -> Sample Control Bus Selector/1
  Sample Control Bus Selector/3 -> General CRC Syndrome Detector HDL Optimized/4
  Sample Control Bus Selector/2 -> General CRC Syndrome Detector HDL Optimized/3
  Sample Control Bus Selector/1 -> General CRC Syndrome Detector HDL Optimized/2
  data_in/1 -> General CRC Syndrome Detector HDL Optimized/1
  General CRC Syndrome Detector HDL Optimized/1 -> data_out/1
  General CRC Syndrome Detector HDL Optimized/2 -> Sample Control Bus Creator/1
  General CRC Syndrome Detector HDL Optimized/3 -> Switch/2, Sample Control Bus Creator/2
  General CRC Syndrome Detector HDL Optimized/4 -> Sample Control Bus Creator/3
  Sample Control Bus Creator/1 -> ctrl_out/1
  Unit Delay/1 -> Switch/3
  Switch/1 -> err/1, Unit Delay/1
  General CRC Syndrome Detector HDL Optimized/5 -> Switch/1

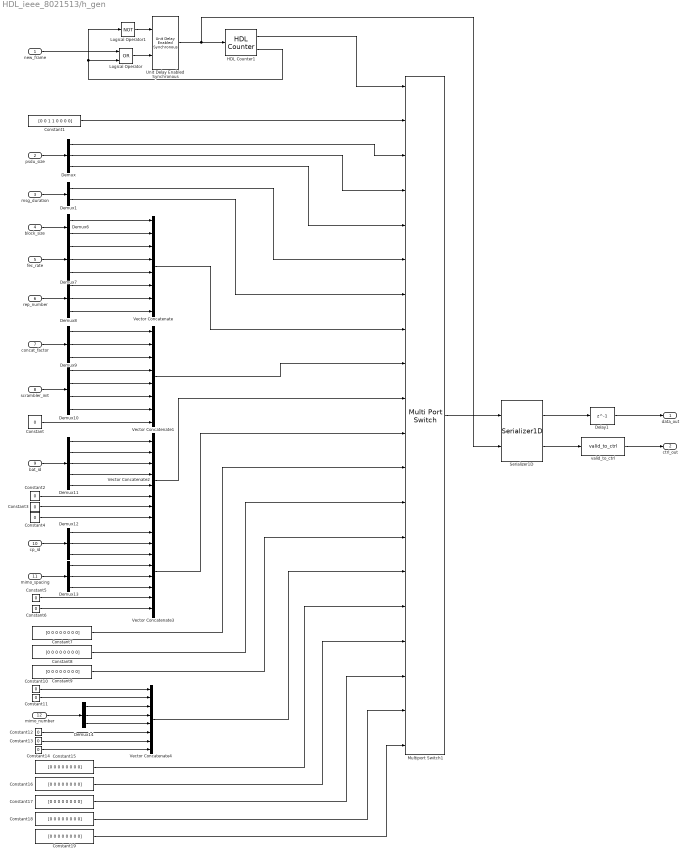
== system HDL_ieee_8021513/h_gen ==
  new_frame : Inport
  psdu_size : Inport  Port=2
  msg_duration : Inport  Port=3
  block_size : Inport  Port=4
  fec_rate : Inport  Port=5
  rep_number : Inport  Port=6
  concat_factor : Inport  Port=7
  scrambler_init : Inport  Port=8
  bat_id : Inport  Port=9
  cp_id : Inport  Port=10
  mimo_spacing : Inport  Port=11
  mimo_number : Inport  Port=12
  Constant{,2..6,10..14} (11 alike) : Constant  Value=0  OutDataTypeStr=boolean  SampleTime=-1
  Constant1 : Constant  Value=[0 0 1 1 0 0 0 0]  VectorParams1D=off  OutDataTypeStr=boolean  SampleTime=-1
  Constant{7..9,15..19} (8 alike) : Constant  Value=[0 0 0 0 0 0 0 0]  VectorParams1D=off  OutDataTypeStr=boolean  SampleTime=-1
  Delay1 : Delay  DelayLength=1  InitialCondition=0  UseCircularBuffer=on
  Demux{,7..9,12..14} (7 alike) : Demux  Outputs=3
  Demux1 : Demux  Outputs=2
  Demux10 : Demux
  Demux11 : Demux  Outputs=5
  Demux6 : Demux  Outputs=2
  HDL Counter1 : hdlsllib/Sources/HDL Counter  CountType=Count limited  CountInit=0  CountStep=1  CountMax=18  CountFromType=Initial value  CountFrom=0  CountResetPort=off  CountLoadPort=off  CountEnbPort=on  CountDirPort=off  CountHitOutputPort=on  CountDataType=Unsigned  CountWordLen=5  CountFracLen=0  CountSampTime=1
  Logical Operator : Logic  Operator=OR  IconShape=distinctive  AllPortsSameDT=off  OutDataTypeStr=boolean
  Logical Operator1 : Logic  Operator=NOT  IconShape=distinctive  AllPortsSameDT=off  OutDataTypeStr=boolean
  Multiport Switch1 : MultiPortSwitch  DataPortOrder=Zero-based contiguous  Inputs=19  zeroidx=on  OutDataTypeStr=Inherit: Same as first data input  SaturateOnIntegerOverflow=off
  Serializer1D : hdlsllib/HDL Operations/Serializer1D  Ratio=8  IdleCycles=0  validIn=on  startOut=off  validOut=on  inputDataDimensions=-1  inputSampleTime=-1  inputSignalType=auto
  Unit Delay Enabled Synchronous : hdlsllib/Discrete/Unit Delay Enabled Synchronous  InitialCondition=0.0  SampleTime=-1
  Vector Concatenate{,1..4} (5 alike) : Concatenate  NumInputs=8  Mode=Multidimensional array  ConcatenateDimension=2
  valid_to_ctrl : $bdroot/valid_to_ctrl  SystemSampleTime=-1  VariantActivationTime=update diagram  AllowFlexibleInterface=on  Latency=0  AutoFrameSizeCalculation=off
  data_out : Outport  VectorParamsAs1DForOutWhenUnconnected=off
  ctrl_out : Outport  Port=2  VectorParamsAs1DForOutWhenUnconnected=off
  wires:
  mimo_number/1 -> Demux14/1
  msg_duration/1 -> Demux1/1
  rep_number/1 -> Demux8/1
  fec_rate/1 -> Demux7/1
  block_size/1 -> Demux6/1
  concat_factor/1 -> Demux9/1
  scrambler_init/1 -> Demux10/1
  Demux/2 -> Multiport Switch1/4
  Demux/3 -> Multiport Switch1/5
  Demux1/2 -> Multiport Switch1/7
  Constant1/1 -> Multiport Switch1/2
  Vector Concatenate/1 -> Multiport Switch1/8
  Constant/1 -> Vector Concatenate1/8
  bat_id/1 -> Demux11/1
  Constant2/1 -> Vector Concatenate2/6
  Constant3/1 -> Vector Concatenate2/7
  Constant4/1 -> Vector Concatenate2/8
  Constant5/1 -> Vector Concatenate3/7
  Constant6/1 -> Vector Concatenate3/8
  Constant10/1 -> Vector Concatenate4/1
  Constant11/1 -> Vector Concatenate4/2
  Constant12/1 -> Vector Concatenate4/6
  Constant13/1 -> Vector Concatenate4/7
  Constant14/1 -> Vector Concatenate4/8
  Vector Concatenate1/1 -> Multiport Switch1/9
  Vector Concatenate2/1 -> Multiport Switch1/10
  Vector Concatenate3/1 -> Multiport Switch1/11
  Constant7/1 -> Multiport Switch1/12
  Constant8/1 -> Multiport Switch1/13
  Constant9/1 -> Multiport Switch1/14
  Vector Concatenate4/1 -> Multiport Switch1/15
  Constant15/1 -> Multiport Switch1/16
  Constant16/1 -> Multiport Switch1/17
  Constant17/1 -> Multiport Switch1/18
  Constant18/1 -> Multiport Switch1/19
  Constant19/1 -> Multiport Switch1/20
  HDL Counter1/1 -> Multiport Switch1/1
  Multiport Switch1/1 -> Serializer1D/1
  Serializer1D/1 -> Delay1/1
  new_frame/1 -> Logical Operator/1
  HDL Counter1/2 -> Logical Operator/2, Logical Operator1/1
  Logical Operator/1 -> Unit Delay Enabled Synchronous/2
  Unit Delay Enabled Synchronous/1 -> Serializer1D/2, HDL Counter1/1
  Logical Operator1/1 -> Unit Delay Enabled Synchronous/1
  Delay1/1 -> data_out/1
  Serializer1D/2 -> valid_to_ctrl/1
  valid_to_ctrl/1 -> ctrl_out/1
  Demux6/1 -> Vector Concatenate/1
  Demux6/2 -> Vector Concatenate/2
  Demux7/1 -> Vector Concatenate/3
  Demux7/2 -> Vector Concatenate/4
  Demux7/3 -> Vector Concatenate/5
  Demux8/1 -> Vector Concatenate/6
  Demux8/2 -> Vector Concatenate/7
  Demux8/3 -> Vector Concatenate/8
  Demux9/1 -> Vector Concatenate1/1
  Demux9/2 -> Vector Concatenate1/2
  Demux9/3 -> Vector Concatenate1/3
  Demux10/1 -> Vector Concatenate1/4
  Demux10/2 -> Vector Concatenate1/5
  Demux10/3 -> Vector Concatenate1/6
  Demux10/4 -> Vector Concatenate1/7
  Demux11/1 -> Vector Concatenate2/1
  Demux11/2 -> Vector Concatenate2/2
  Demux11/3 -> Vector Concatenate2/3
  Demux11/4 -> Vector Concatenate2/4
  Demux11/5 -> Vector Concatenate2/5
  Demux12/1 -> Vector Concatenate3/1
  Demux12/2 -> Vector Concatenate3/2
  Demux12/3 -> Vector Concatenate3/3
  Demux13/1 -> Vector Concatenate3/4
  Demux13/2 -> Vector Concatenate3/5
  Demux13/3 -> Vector Concatenate3/6
  Demux14/1 -> Vector Concatenate4/3
  Demux14/2 -> Vector Concatenate4/4
  Demux14/3 -> Vector Concatenate4/5
  psdu_size/1 -> Demux/1
  cp_id/1 -> Demux12/1
  mimo_spacing/1 -> Demux13/1
  Demux/1 -> Multiport Switch1/3
  Demux1/1 -> Multiport Switch1/6

== system HDL_ieee_8021513/h_remove_repetition ==
  data_in : Inport
  start_in : Inport  Port=2
  HDL Counter : hdlsllib/Sources/HDL Counter  CountType=Count limited  CountInit=0  CountStep=1  CountMax=headerBitsPerFec-1  CountFromType=Initial value  CountFrom=0  CountResetPort=on  CountLoadPort=off  CountEnbPort=on  CountDirPort=off  CountHitOutputPort=on  CountDataType=Unsigned  CountWordLen=nextpow2(headerBitsPerFec)  CountFracLen=0  CountSampTime=1
  Logical Operator : Logic  Operator=OR  AllPortsSameDT=off  OutDataTypeStr=boolean
  Sample Control Bus Creator : whdlutilities/Sample Control Bus Creator
  Switch : Switch  Criteria=u2 ~= 0  SaturateOnIntegerOverflow=off  InputSameDT=off
  Terminator : Terminator
  Unit Delay{,1..7} (8 alike) : UnitDelay  SampleTime=-1  HasFrameUpgradeWarning=on
  data_out : Outport
  ctrl_out : Outport  Port=2
  wires:
  start_in/1 -> Unit Delay3/1, Logical Operator/1, Unit Delay2/1
  HDL Counter/2 -> Logical Operator/2, Sample Control Bus Creator/2
  data_in/1 -> Unit Delay4/1
  Sample Control Bus Creator/1 -> ctrl_out/1
  Unit Delay/1 -> Switch/3
  HDL Counter/1 -> Terminator/1  "count"
  Logical Operator/1 -> Unit Delay1/1
  Unit Delay1/1 -> Switch/2
  Unit Delay2/1 -> Switch/1
  Unit Delay4/1 -> Unit Delay5/1  "data_in"
  Unit Delay3/1 -> Unit Delay6/1, HDL Counter/1  "rst"
  Switch/1 -> Unit Delay7/1, HDL Counter/2, Unit Delay/1
  Unit Delay5/1 -> data_out/1
  Unit Delay6/1 -> Sample Control Bus Creator/1
  Unit Delay7/1 -> Sample Control Bus Creator/3

== system HDL_ieee_8021513/h_repetition ==
  data_in : Inport
  ctrl_in : Inport  Port=2
  Bus Selector : BusSelector  OutputSignals=start,end,valid
  Delay{,1..4} (5 alike) : Delay  DelayLength=1  InitialCondition=0  UseCircularBuffer=on
  HDL Counter2 : hdlsllib/Sources/HDL Counter  CountType=Count limited  CountInit=headerBitsPerFec-2  CountStep=1  CountMax=headerBitsPerFec-1  CountFromType=Specify  CountFrom=0  CountResetPort=off  CountLoadPort=off  CountEnbPort=on  CountDirPort=off  CountHitOutputPort=off  CountDataType=Unsigned  CountWordLen=nextpow2(headerBitsPerOFDMSymbol)  CountFracLen=0  CountSampTime=1
  HDL Counter3 : hdlsllib/Sources/HDL Counter  CountType=Count limited  CountInit=0  CountStep=1  CountMax=headerBitsPerOFDMSymbol - headerBitsPerFec -1  CountFromType=Initial value  CountFrom=0  CountResetPort=off  CountLoadPort=off  CountEnbPort=on  CountDirPort=off  CountHitOutputPort=on  CountDataType=Unsigned  CountWordLen=nextpow2(headerBitsPerOFDMSymbol)  CountFracLen=0  CountSampTime=1
  Logical Operator : Logic  Operator=NOT  IconShape=distinctive  AllPortsSameDT=off  OutDataTypeStr=boolean
  Logical Operator1 : Logic  Operator=OR  IconShape=distinctive  AllPortsSameDT=off  OutDataTypeStr=boolean
  Logical Operator2 : Logic  Operator=NOT  IconShape=distinctive  AllPortsSameDT=off  OutDataTypeStr=boolean
  NOT : Logic  Operator=NOT  IconShape=distinctive  AllPortsSameDT=off  OutDataTypeStr=boolean
  Sample Control Bus Creator : whdlutilities/Sample Control Bus Creator
  Simple Dual Port RAM : hdlsllib/HDL RAMs/Simple Dual Port RAM  ram_size=nextpow2(headerBitsPerOFDMSymbol)
  Switch : Switch  Criteria=u2 ~= 0  SaturateOnIntegerOverflow=off  InputSameDT=off
  Switch1 : Switch  Criteria=u2 ~= 0  SaturateOnIntegerOverflow=off  InputSameDT=off
  Unit Delay Enabled Synchronous1 : hdlsllib/Discrete/Unit Delay Enabled Synchronous  InitialCondition=0.0  SampleTime=-1
  data_out : Outport  VectorParamsAs1DForOutWhenUnconnected=off
  ctrl_out : Outport  Port=2  VectorParamsAs1DForOutWhenUnconnected=off
  wires:
  Delay4/1 -> [end_out]
  Delay3/1 -> Switch1/1
  ctrl_in/1 -> Bus Selector/1
  Bus Selector/3 -> [valid], Delay3/1  "<valid>"
  Sample Control Bus Creator/1 -> ctrl_out/1
  Bus Selector/1 -> Delay/1  "<start>"
  Bus Selector/2 -> [end]  "<end>"
  Delay/1 -> Sample Control Bus Creator/1
  [end_out] -> Sample Control Bus Creator/2
  Switch1/1 -> Sample Control Bus Creator/3
  [valid] -> HDL Counter2/1  "addrB_valid"
  [valid] -> Simple Dual Port RAM/3
  HDL Counter2/1 -> Simple Dual Port RAM/2
  data_in/1 -> Delay1/1, Simple Dual Port RAM/1  "datain"
  HDL Counter3/1 -> Simple Dual Port RAM/4  "addrA"
  Unit Delay Enabled Synchronous1/1 -> HDL Counter3/1, Delay2/1
  [end] -> Logical Operator1/1
  Logical Operator1/1 -> Unit Delay Enabled Synchronous1/2
  HDL Counter3/2 -> Logical Operator1/2, NOT/1, Delay4/1
  NOT/1 -> Unit Delay Enabled Synchronous1/1
  Switch/1 -> data_out/1
  Delay2/1 -> Logical Operator2/1, Switch1/3, Logical Operator/1
  Simple Dual Port RAM/1 -> Switch/3
  Delay1/1 -> Switch/1
  Logical Operator/1 -> Switch1/2
  Logical Operator2/1 -> Switch/2

== system HDL_ieee_8021513/h_rx_full ==
  data_in : Inport
  start_in : Inport  Port=2
  Data Type Conversion : DataTypeConversion  OutDataTypeStr=int8  SaturateOnIntegerOverflow=off  RndMeth=Floor
  Data Type Conversion1 : DataTypeConversion  OutDataTypeStr=boolean  SaturateOnIntegerOverflow=off  RndMeth=Floor
  LDPC_Deco_Hc_12H : whdledac/LDPC Decoder  ParityCheckMatrix=Hc_12H  BlockSize=14  Algorithm=Min-sum  ScalingFactor=0.75  Termination=Max  SpecifyInputs=Property  NumIterations=ldpcDecoderMaxNumberIterations  MaxNumIterations=8  ParityCheckStatus=off  SimulateUsing=Code generation
  Rate Transition : RateTransition  OutPortSampleTimeOpt=Multiple of input port sample time  OutPortSampleTimeMultiple=8
  Terminator : Terminator
  h_crc_rx : $bdroot/h_crc_rx  SystemSampleTime=-1  VariantActivationTime=update diagram  AllowFlexibleInterface=on  Latency=0  AutoFrameSizeCalculation=off
  h_remove_repetition : $bdroot/h_remove_repetition  SystemSampleTime=-1  VariantActivationTime=update diagram  AllowFlexibleInterface=on  Latency=0  AutoFrameSizeCalculation=off
  h_scrambler : $bdroot/h_scrambler  SystemSampleTime=-1  VariantActivationTime=update diagram  AllowFlexibleInterface=on  Latency=0  AutoFrameSizeCalculation=off
      settings: LibrarySourceBlock=|
      | hdlsllib/Ports &
      | Subsystems/Subsystem
  h_separate : $bdroot/h_separate  SystemSampleTime=-1  VariantActivationTime=update diagram  AllowFlexibleInterface=on  Latency=0  AutoFrameSizeCalculation=off
  psdu_size : Outport
  msg_duration : Outport  Port=2
  block_size : Outport  Port=3
  fec_rate : Outport  Port=4
  rep_number : Outport  Port=5
  concat_factor : Outport  Port=6
  scrambler_init : Outport  Port=7
  bat_id : Outport  Port=8
  cp_id : Outport  Port=9
  mimo_spacing : Outport  Port=10
  mimo_number : Outport  Port=11
  end : Outport  Port=12
  err : Outport  Port=13
  wires:
  Rate Transition/1 -> err/1
  h_separate/4 -> fec_rate/1
  h_separate/1 -> psdu_size/1
  h_remove_repetition/2 -> LDPC_Deco_Hc_12H/2
  LDPC_Deco_Hc_12H/2 -> h_scrambler/2
  h_crc_rx/2 -> h_separate/2
  h_scrambler/2 -> h_crc_rx/2
  h_separate/7 -> scrambler_init/1
  h_scrambler/1 -> h_crc_rx/1
  h_separate/5 -> rep_number/1
  h_separate/11 -> mimo_number/1
  h_crc_rx/1 -> h_separate/1
  h_separate/9 -> cp_id/1
  h_crc_rx/3 -> Rate Transition/1
  start_in/1 -> Data Type Conversion1/1
  LDPC_Deco_Hc_12H/1 -> h_scrambler/1
  h_separate/8 -> bat_id/1
  data_in/1 -> Data Type Conversion/1
  h_remove_repetition/1 -> LDPC_Deco_Hc_12H/1
  h_separate/2 -> msg_duration/1
  h_separate/10 -> mimo_spacing/1
  LDPC_Deco_Hc_12H/3 -> Terminator/1
  h_separate/6 -> concat_factor/1
  h_separate/12 -> end/1
  h_separate/3 -> block_size/1
  Data Type Conversion/1 -> h_remove_repetition/1
  Data Type Conversion1/1 -> h_remove_repetition/2
